simulink model "controlo_atitude_GulfVsim"  (R2020b)
settings: Solver=VariableStepAuto  StartTime=0.0  StopTime=100  RelTol=1e-3
values from neighbouring files (symbols this model uses):
  a = [ ... (first row only)    [espaco_estados_GulfV.m]
  b = [ ... (first row only)    [espaco_estados_GulfV.m]
  F = inv(G)    [controlo_atitude_GulfV.m]
  k_lqr = lqr(a,b,q,r)    [controlo_atitude_GulfV.m]
settings Model: Creator=Admin  LastModifiedBy=Admin

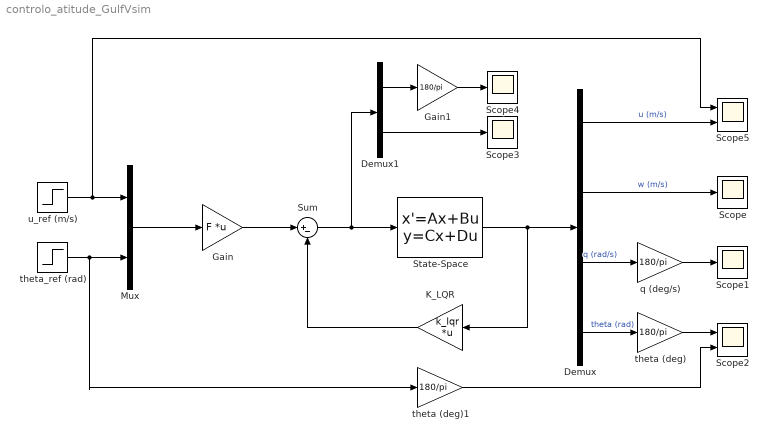
== system controlo_atitude_GulfVsim ==
  Demux : Demux
  Demux1 : Demux  Outputs=2
  Gain : Gain  Gain=F  Multiplication=Matrix(K*u)
  Gain1 : Gain  Gain=180/pi
  K_LQR : Gain  Gain=k_lqr  Multiplication=Matrix(K*u)
  Mux : Mux  Inputs=2
  Scope{,1,3..4} (4 alike) : Scope
  Scope2 : Scope  NumInputPorts=2
  Scope5 : Scope  NumInputPorts=2
  State-Space : StateSpace  A=a  B=b  C=eye(4)  D=zeros(4,2)  InitialCondition=0
  Sum : Sum  Inputs=|+-
  q (deg/s) : Gain  Gain=180/pi
  theta (deg) : Gain  Gain=180/pi
  theta (deg)1 : Gain  Gain=180/pi
  theta_ref (rad) : Step  Time=5  After=0.0873  SampleTime=0
  u_ref (m/s) : Step  Time=50  After=2  SampleTime=0
  wires:
  State-Space/1 -> K_LQR/1, Demux/1
  Demux/1 -> Scope5/2  "u (m/s)"
  Demux/2 -> Scope/1  "w (m/s)"
  Demux/3 -> q (deg/s)/1  "q (rad/s)"
  Demux/4 -> theta (deg)/1  "theta (rad)"
  q (deg/s)/1 -> Scope1/1
  theta (deg)/1 -> Scope2/1
  Sum/1 -> Demux1/1, State-Space/1
  K_LQR/1 -> Sum/2
  Gain/1 -> Sum/1
  Mux/1 -> Gain/1
  theta_ref (rad)/1 -> theta (deg)1/1, Mux/2
  Demux1/2 -> Scope3/1
  Demux1/1 -> Gain1/1
  u_ref (m/s)/1 -> Scope5/1, Mux/1
  theta (deg)1/1 -> Scope2/2
  Gain1/1 -> Scope4/1
